simulink model "Trab1_desafio_4_f"  (R2018a)
settings: Solver=VariableStepAuto  StartTime=0.0  StopTime=10.0  RelTol=1e-4
values from neighbouring files (symbols this model uses):
  A22 = Ad(k+1:end,k+1:end)    [Trab1_desafio4.m]
  B2 = Bd(k+1:end,:)    [Trab1_desafio4.m]
  C2 = Cd(:,k+1:end)    [Trab1_desafio4.m]
  invWo = inv(obsv_gramm(A22,C2,Tf))    [Trab1_desafio4.m]
  Tf = 5    [Trab1_desafio4.m]
  z0_obs = z0(k+1:end,1)    [Trab1_desafio4.m]
undefined symbols (not defined in the file or in its folder): calc_expm
settings Model: Creator=eric-  LastModifiedBy=eric-

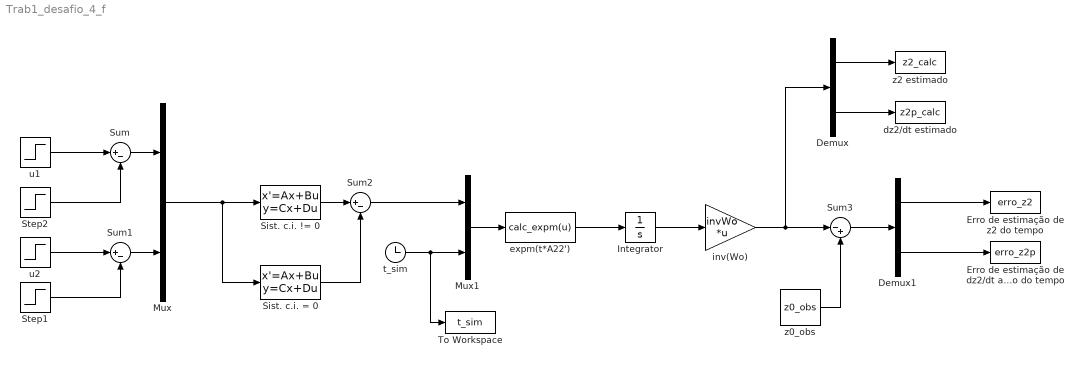
== system Trab1_desafio_4_f ==
  Demux : Demux  Outputs=2
  Demux1 : Demux  Outputs=2
  Erro de estimação de dz2/dt ao longo do tempo : ToWorkspace  VariableName=erro_z2p  SampleTime=-1
      settings: Save2DSignal=2-D array (concatenate along first dimension)
  Erro de estimação de z2 do tempo : ToWorkspace  VariableName=erro_z2  SampleTime=-1
      settings: Save2DSignal=2-D array (concatenate along first dimension)
  Integrator : Integrator
  Mux : Mux  Inputs=2
  Mux1 : Mux  Inputs=2
  Sist. c.i. != 0 : StateSpace  A=A22  B=B2  C=C2  D=[0 0]  InitialCondition=z0_obs
  Sist. c.i. = 0 : StateSpace  A=A22  B=B2  C=C2  D=[0 0]  InitialCondition=[0;0]
  Step1 : Step  Time=Tf  SampleTime=0
  Step2 : Step  Time=Tf  SampleTime=0
  Sum : Sum  Inputs=|+-
  Sum1 : Sum  Inputs=|+-
  Sum2 : Sum  Inputs=|+-
  Sum3 : Sum  Inputs=|-+
  To Workspace : ToWorkspace  VariableName=t_sim  SampleTime=-1
      settings: Save2DSignal=2-D array (concatenate along first dimension)
  dz2/dt estimado : ToWorkspace  VariableName=z2p_calc  SampleTime=-1
      settings: Save2DSignal=2-D array (concatenate along first dimension)
  expm(t*A22') : MATLABFcn  MATLABFcn=calc_expm(u)
  inv(Wo) : Gain  Gain=invWo  Multiplication=Matrix(K*u)
  t_sim : Clock
  u1 : Step  Time=0  SampleTime=0
  u2 : Step  Time=0  SampleTime=0
  z0_obs : Constant  Value=z0_obs
  z2 estimado : ToWorkspace  VariableName=z2_calc  SampleTime=-1
      settings: Save2DSignal=2-D array (concatenate along first dimension)
  wires:
  Mux/1 -> Sist. c.i. = 0/1, Sist. c.i. != 0/1
  u1/1 -> Sum/1
  Step2/1 -> Sum/2
  Sum/1 -> Mux/1
  u2/1 -> Sum1/1
  Sum1/1 -> Mux/2
  Step1/1 -> Sum1/2
  Sist. c.i. != 0/1 -> Sum2/1
  Sist. c.i. = 0/1 -> Sum2/2
  Sum2/1 -> Mux1/1
  t_sim/1 -> To Workspace/1, Mux1/2
  Mux1/1 -> expm(t*A22')/1
  expm(t*A22')/1 -> Integrator/1
  z0_obs/1 -> Sum3/2
  Integrator/1 -> inv(Wo)/1
  inv(Wo)/1 -> Demux/1, Sum3/1
  Demux/1 -> z2 estimado/1
  Demux/2 -> dz2/dt estimado/1
  Sum3/1 -> Demux1/1
  Demux1/2 -> Erro de estimação de dz2/dt ao longo do tempo/1
  Demux1/1 -> Erro de estimação de z2 do tempo/1
